simulink model "MotorSimu"  (R2023b)
settings: Solver=VariableStepAuto  StartTime=0.0  StopTime=10.0  RelTol=1e-3
undefined symbols (not defined in the file): b, J, Ke, Kt, L, R
settings Model: Creator=USER  LastModifiedBy=USER

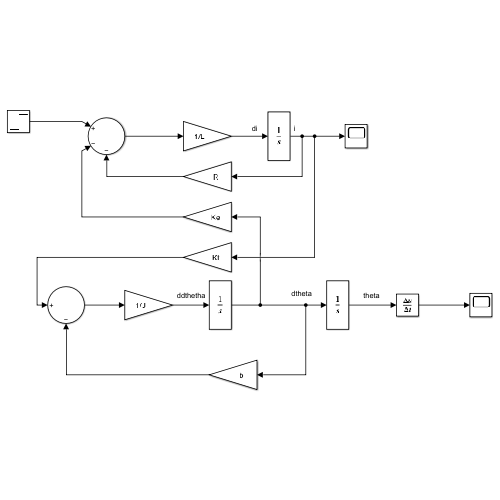
[thumbnail: Simulink's stored preview of the top-level diagram]
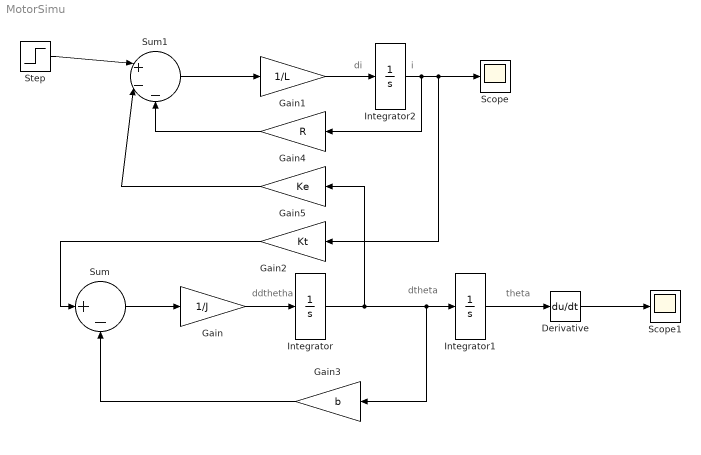
== system MotorSimu ==
  note: di
  note: theta
  note: dtheta
  note: ddthetha
  note: i
  Derivative : Derivative
  Gain : Gain  Gain=1/J
  Gain1 : Gain  Gain=1/L
  Gain2 : Gain  Gain=Kt
  Gain3 : Gain  Gain=b
  Gain4 : Gain  Gain=R
  Gain5 : Gain  Gain=Ke
  Integrator : Integrator
  Integrator1 : Integrator
  Integrator2 : Integrator
  Scope : Scope
  Scope1 : Scope
  Step : Step  Time=0  After=5  SampleTime=0
  Sum : Sum  Inputs=|+-
  Sum1 : Sum  Inputs=|+--
  wires:
  Integrator/1 -> Gain5/1, Gain3/1, Integrator1/1
  Gain/1 -> Integrator/1
  Sum/1 -> Gain/1
  Gain1/1 -> Integrator2/1
  Sum1/1 -> Gain1/1
  Integrator1/1 -> Derivative/1
  Integrator2/1 -> Gain4/1, Gain2/1, Scope/1
  Gain2/1 -> Sum/1
  Gain3/1 -> Sum/2
  Step/1 -> Sum1/1
  Gain4/1 -> Sum1/3
  Gain5/1 -> Sum1/2
  Derivative/1 -> Scope1/1
